simulink model "rlQubeServo"  (R2024a)
settings: Solver=ode23t  StartTime=0.0  StopTime=10.0  RelTol=1e-3  AbsTol=1e-3
values from neighbouring files (symbols this model uses):
  D_p = 8e-6    (= 8e-06)    [loadQubeParameters.m]
  D_r_2 = 1.88e-04    (= 0.000188)    [loadQubeParameters.m]
  dphi0 = 0    [loadQubeParameters.m]
  dphi_gain = 2    [loadQubeParameters.m]
  dtheta0 = 0    [loadQubeParameters.m]
  dtheta_gain = 0.0356    [loadQubeParameters.m]
  K_b_2 = 0.182    [loadQubeParameters.m]
  K_t = 0.042    [loadQubeParameters.m]
  L_m = 4.98e-3    (= 0.00498)    [loadQubeParameters.m]
  L_p = 0.126    [loadQubeParameters.m]
  L_r = 0.103    [loadQubeParameters.m]
  m_p = 0.024    [loadQubeParameters.m]
  m_r = 0.095    [loadQubeParameters.m]
  mu_m = 3.08e-6    (= 3.08e-06)    [loadQubeParameters.m]
  n = 1    [loadQubeParameters.m]
  p_rad = 0.0045    [loadQubeParameters.m]
  phi0 = 0    [loadQubeParameters.m]
  phi_gain = 40    [loadQubeParameters.m]
  R_m = 21.7    [loadQubeParameters.m]
  rod_rad = 0.003    [loadQubeParameters.m]
  Tf = 10    [loadQubeParameters.m]
  theta0 = 0    [loadQubeParameters.m]
  theta_gain = 0.162    [loadQubeParameters.m]
  Ts = Tc * 4    (= 0.02)    [loadQubeParameters.m]
  Volt_Limit = 12    [loadQubeParameters.m]
undefined symbols (not defined in the file or in its folder): X, Y, Z
libraries: sm_lib x21, fl_lib x10, nesl_utility x9, rllib x2, simulink x2, ee_lib x1
(part 1 of 2)
settings Model: Creator=The MathWorks, Inc.  LastModifiedBy=niels
settings SolverCC: AutoScaleAbsTol=off  MaxZcPerStep=1
settings DebuggingCC: UnconnectedInputMsg=warning  UnconnectedOutputMsg=warning  UnconnectedLineMsg=warning
settings ModelReferenceCC: EnableRefExpFcnMdlSchedulingChecks=on
settings RTWCC: GPUComputeCapability=3.5  DLArmComputeVersion=19.05
settings ExplorerConfigSet: InternalSimMechanicsExplorerSettings="<ExplorerConfiguration><canonicalview>default</canonicalview><AnimationSetting><BasePlaybackSpeed>1.0</BasePlaybackSpeed><PlaybackSpeedFactor>1.0</PlaybackSpeedFactor></AnimationSetting><TilePanel><TileInfo><Tiles Columns=\"1\" Count=\"1\" Rows=\"1\"><Column Weight=\"1\"/><Row Weight=\"1\"/><Tile Height=\"1\" Width=\"1\" X=\"0\" Y=\"0\"/></Tiles></TileInfo><SceneInfo><SceneViewer><BGColor><R>0.60000002384185791</R><G>0.60000002384185791</G><B>0.60000002384185791</B></BGColor><Camera><DoPerspective>on</DoPerspective><Position><X>0.334156231583514596</X><Y>0.107146061295956732</Y><Z>0.154419804164132285</Z></Position><Center><X>0.145480827141795971</X><Y>0.0537418892551446009</Y><Z>0.077934111254939889</Z></Center><Up><X>-0.332530024195597795</X><Y>-0.157027945704575345</Y><Z>0.929927958110882913</Z></Up><ViewLimDist>1</ViewLimDist><YLim>0.466307658154998583</YLim><XLim>0.535390274177961367</XLim></Camera></SceneViewer></SceneInfo></TilePanel><MechEditorPanel><Cameras><Camera><Id>Camera1</Id><Value><Name>Camera1</Name><NativeCamera><PositionKeyframeSet/><CenterKeyframeSet/><UpVectorKeyframeSet/></NativeCamera></Value></Camera></Cameras><GfxPanelCameraMap><MapElement CameraMLId=\"Camera1\" GfxPanelIndex=\"0\"/></GfxPanelCameraMap><VideoCreator><PlaybackSpeedRatio>1.0</PlaybackSpeedRatio><FrameRate>30</FrameRate><VideoFormat>Motion JPEG AVI</VideoFormat><FrameSize>auto</FrameSize></VideoCreator></MechEditorPanel></ExplorerConfiguration>"

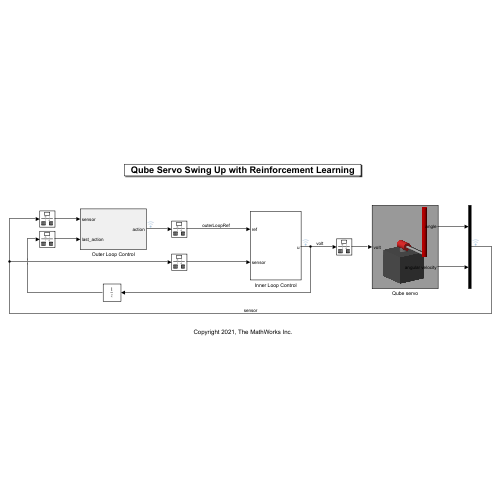
[thumbnail: Simulink's stored preview of the top-level diagram]
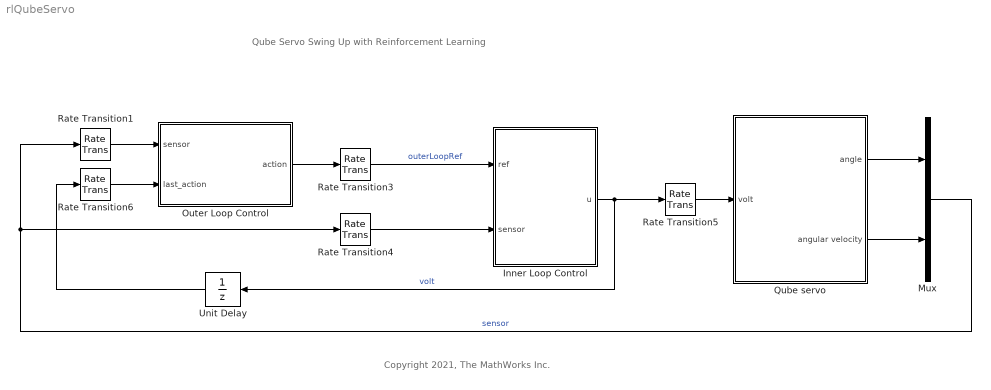
== system rlQubeServo ==
  note: Qube Servo Swing Up with Reinforcement Learning
  note: Copyright 2021, The MathWorks Inc.
  Inner Loop Control : Subsystem
  Mux : Mux  Inputs=2
  Outer Loop Control : Subsystem  mask{DesignModeChoice=Mode select}
      mask prompts: DesignModeChoice "Design mode"
      mask init:
      | choice = get_param(gcb,'DesignModeChoice');
      | vssBlk = [gcb,'/RL_Mode_Select/Variant Source'];
      | if strcmp(choice,'Swing up')
      |     set_param(vssBlk, 'LabelModeActiveChoice', 'RL_DESIGN_MODE_SWING_UP');
      | else
      |     set_param(vssBlk, 'LabelModeActiveChoice', 'RL_DESIGN_MODE_SELECT_MODE');
      | end
      mask TypeOptions DesignModeChoice: Mode select | Swing up
      mask DialogControl DescGroupVar Prompt: Description
      mask DialogControl DescTextVar Prompt: Select a design mode for the planner.
      mask DialogControl Control4 Prompt: A) Mode select:
      mask DialogControl Control2 Prompt: Select reference signal source for either pendulum swing up or balancing.
      mask DialogControl Control5 Prompt: B) Swing up:
      mask DialogControl Control3 Prompt: Swing up the pendulum from stable equilibrium position (phi=0 deg) without balancing
  Qube servo : Subsystem  mask(Qube servo 2 model by Simscape){a0=[theta0, phi0], w0=[dtheta0, dphi0], R_m=R_m, L_m=L_m, mu_m=mu_m, K_b=K_b_2, n=n, rod_mass=m_r, rod_length=L_r, rod_rad=rod_rad, p_mass=m_p, p_length=L_p, p_rad=p_rad, D_r=D_r_2, D_p=D_p, Choice_Stopper=Off}
      mask prompts: a0 "Init angle (theta phi) [rad]"; w0 "Init velocity (theta_dot phi_dot) [rad/s]"; R_m "Motor Resistance of [Ohm]"; L_m "Motor Inductance [H]"; mu_m "Motor Damping [Nm/rad/s]"; K_b "Back EMF contant [V/(rad/s)]"; n "Gear Ratio [-]"; rod_mass "Mass of Arm rod [kg]"; rod_length "Length of Arm rod [m]"; rod_rad "Radius of Arm rod [m]"; p_mass "Mass of Pendulum [kg]"; p_length "Length of Pendulum [m]"; p_rad "Radius of Pendulum [m]"; D_r "Damping of Arm rod [Nm/rad/s]"; D_p "Damping of Pendulum [Nm/rad/s]"; Choice_Stopper "Servo stopper"
      mask init:
      | % Density [kg/m^3] of each component
      | rho_rod = rod_mass/(pi*rod_rad^2*rod_length);
      | rho_p = p_mass/(pi*p_rad^2*p_length);
      | 
      | choice = get_param(gcb,'Choice_Stopper');
      | vssBlk = [gcb,'/Pendulum Physical Model/stopper'];
      | if strcmp(choice,'Off')
      |     set_param(vssBlk, 'LabelModeActiveChoice', 'Choice_Qube_Stopper_Off');
      | else
      |     set_param(vssBlk, 'LabelModeActiveChoice', 'Choice_Qube_Stopper_On');
      | end
      mask TypeOptions Choice_Stopper: Off | On
      mask DialogControl Container4 Prompt: Inital Conditions
      mask DialogControl Container3 Prompt: Parameters
      mask DialogControl Container7 Prompt: Options
      mask Display: image('$imagefile'); % Use "Edit Image" on toolstrip to change.
  Rate Transition1 : RateTransition  OutPortSampleTime=Ts
  Rate Transition3 : RateTransition  OutPortSampleTime=Tc
  Rate Transition4 : RateTransition  OutPortSampleTime=Tc
  Rate Transition5 : RateTransition
  Rate Transition6 : RateTransition  OutPortSampleTime=Ts
  Unit Delay : UnitDelay  SampleTime=-1  HasFrameUpgradeWarning=on
  wires:
  Qube servo/1(angle) -> Mux/1
  Qube servo/2(angular velocity) -> Mux/2
  Rate Transition4/1 -> Inner Loop Control/2(sensor)
  Inner Loop Control/1(u) -> Rate Transition5/1, Unit Delay/1  "volt"
  Rate Transition5/1 -> Qube servo/1(volt)
  Rate Transition3/1 -> Inner Loop Control/1(ref)  "outerLoopRef"
  Mux/1 -> Rate Transition1/1, Rate Transition4/1  "sensor"
  Unit Delay/1 -> Rate Transition6/1
  Rate Transition1/1 -> Outer Loop Control/1(sensor)
  Rate Transition6/1 -> Outer Loop Control/2(last_action)
  Outer Loop Control/1(action) -> Rate Transition3/1

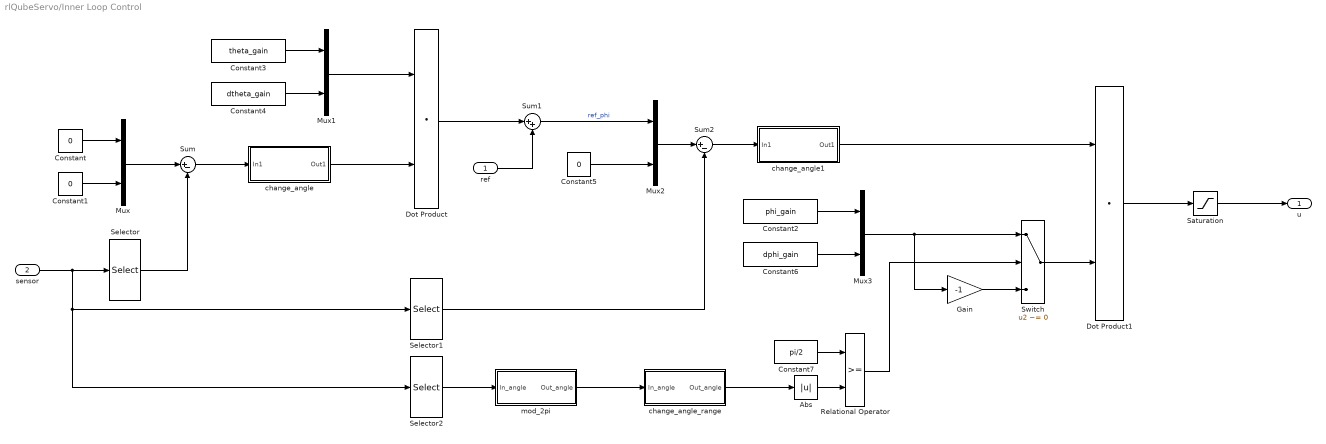
== system rlQubeServo/Inner Loop Control ==
  ref : Inport
  sensor : Inport  Port=2  PortDimensions=4
  Abs : Abs  SaturateOnIntegerOverflow=off
  Constant : Constant  Value=0
  Constant1 : Constant  Value=0
  Constant2 : Constant  Value=phi_gain
  Constant3 : Constant  Value=theta_gain
  Constant4 : Constant  Value=dtheta_gain
  Constant5 : Constant  Value=0
  Constant6 : Constant  Value=dphi_gain
  Constant7 : Constant  Value=pi/2
  Dot Product : DotProduct  OutDataTypeStr=Inherit: Inherit via internal rule
  Dot Product1 : DotProduct  OutDataTypeStr=Inherit: Inherit via internal rule
  Gain : Gain  Gain=-1
  Mux{,1..3} (4 alike) : Mux  Inputs=2
  Relational Operator : RelationalOperator  OutDataTypeStr=boolean  RndMeth=Simplest  InputSameDT=off
  Saturation : Saturate  UpperLimit=Volt_Limit  LowerLimit=-Volt_Limit
  Selector : Selector  InputPortWidth=4  IndexOptions=Index vector (dialog)  Indices=[1 3]  OutputSizes=1
  Selector1 : Selector  InputPortWidth=4  IndexOptions=Index vector (dialog)  Indices=[2 4]  OutputSizes=1
  Selector2 : Selector  InputPortWidth=4  IndexOptions=Index vector (dialog)  Indices=[2]  OutputSizes=1
  Sum : Sum  Inputs=|+-
  Sum1 : Sum  Inputs=|++
  Sum2 : Sum  Inputs=|+-
  Switch : Switch  Criteria=u2 ~= 0  SaturateOnIntegerOverflow=off  InputSameDT=off
  change_angle : Subsystem
  change_angle1 : Subsystem
  change_angle_range : Subsystem
  mod_2pi : Subsystem
  u : Outport
  wires:
  change_angle_range/1(Out_angle) -> Abs/1
  Constant4/1 -> Mux1/2
  Constant2/1 -> Mux3/1
  Saturation/1 -> u/1
  Relational Operator/1 -> Switch/2
  Gain/1 -> Switch/3
  Constant7/1 -> Relational Operator/1
  sensor/1 -> Selector2/1, Selector1/1, Selector/1
  Sum/1 -> change_angle/1(In1)
  ref/1 -> Sum1/2
  Selector1/1 -> Sum2/2
  Selector2/1 -> mod_2pi/1(In_angle)
  Dot Product1/1 -> Saturation/1
  Sum2/1 -> change_angle1/1(In1)
  Constant5/1 -> Mux2/2
  Constant6/1 -> Mux3/2
  Mux2/1 -> Sum2/1
  Abs/1 -> Relational Operator/2
  mod_2pi/1(Out_angle) -> change_angle_range/1(In_angle)
  Sum1/1 -> Mux2/1  "ref_phi"
  Mux1/1 -> Dot Product/1
  Constant3/1 -> Mux1/1
  change_angle1/1(Out1) -> Dot Product1/1
  Constant/1 -> Mux/1
  Dot Product/1 -> Sum1/1
  Mux/1 -> Sum/1
  Mux3/1 -> Switch/1, Gain/1
  Switch/1 -> Dot Product1/2
  Constant1/1 -> Mux/2
  change_angle/1(Out1) -> Dot Product/2
  Selector/1 -> Sum/2

== system rlQubeServo/Outer Loop Control ==
  sensor : Inport
  last_action : Inport  Port=2
  RL_Mode_Select : Subsystem
  RL_Swing_Up : Subsystem
  Switch_Action : Subsystem
  action : Outport
  wires:
  RL_Swing_Up/1(swing_up) -> Switch_Action/2(swing_up)  "action_RL_swing_up"
  Switch_Action/1(out_action) -> action/1  "action"
  sensor/1 -> RL_Swing_Up/1(sensor), RL_Mode_Select/1(sensor)
  RL_Mode_Select/1(select_mode) -> Switch_Action/1(select_mode)  "action_RL_select_mode"
  last_action/1 -> RL_Mode_Select/2(controller_action), RL_Swing_Up/2(controller_action)

== system rlQubeServo/Qube servo ==
  volt : Inport
  DC Motor model : Subsystem
  Pendulum Physical Model : Subsystem
  Terminator1 : Terminator
  angle : Outport
  angular velocity : Outport  Port=2
  wires:
  Pendulum Physical Model/3(Load trq) -> Terminator1/1
  Pendulum Physical Model/1(angle) -> angle/1
  volt/1 -> DC Motor model/1(volt)
  Pendulum Physical Model/2(velocity) -> angular velocity/1
  connections:
  DC Motor model/RConn2 -- Pendulum Physical Model/LConn2
  DC Motor model/RConn1 -- Pendulum Physical Model/LConn1

== system rlQubeServo/Inner Loop Control/change_angle ==
  In1 : Inport
  Demux : Demux  Outputs=2
  Mux : Mux  Inputs=2
  change_angle_range : Subsystem
  mod_2pi : Subsystem
  Out1 : Outport
  wires:
  In1/1 -> Demux/1
  Demux/1 -> mod_2pi/1(In_angle)
  mod_2pi/1(Out_angle) -> change_angle_range/1(In_angle)
  change_angle_range/1(Out_angle) -> Mux/1
  Demux/2 -> Mux/2
  Mux/1 -> Out1/1

== system rlQubeServo/Inner Loop Control/change_angle1 ==
  In1 : Inport
  Demux : Demux  Outputs=2
  Mux : Mux  Inputs=2
  change_angle_range : Subsystem
  mod_2pi : Subsystem
  Out1 : Outport
  wires:
  Mux/1 -> Out1/1
  Demux/2 -> Mux/2
  change_angle_range/1(Out_angle) -> Mux/1
  mod_2pi/1(Out_angle) -> change_angle_range/1(In_angle)
  Demux/1 -> mod_2pi/1(In_angle)
  In1/1 -> Demux/1

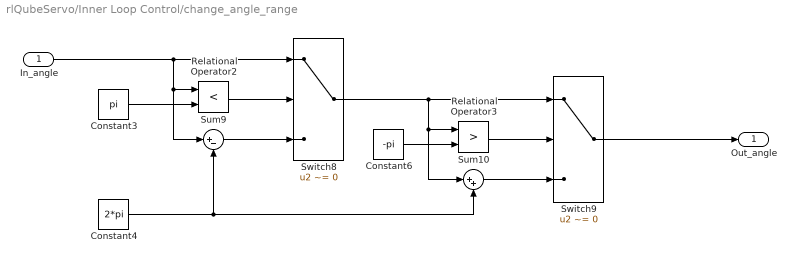
== system rlQubeServo/Inner Loop Control/change_angle_range ==
  In_angle : Inport
  Constant3 : Constant  Value=pi  OutDataTypeStr=Inherit: Inherit via back propagation
  Constant4 : Constant  Value=2*pi  OutDataTypeStr=Inherit: Inherit via back propagation
  Constant6 : Constant  Value=-pi  OutDataTypeStr=Inherit: Inherit via back propagation
  Relational Operator2 : RelationalOperator  Operator=<  OutDataTypeStr=boolean  InputSameDT=off
  Relational Operator3 : RelationalOperator  Operator=>  OutDataTypeStr=boolean  InputSameDT=off
  Sum10 : Sum  Inputs=|++
  Sum9 : Sum  Inputs=|+-
  Switch8 : Switch  Criteria=u2 ~= 0  SaturateOnIntegerOverflow=off  InputSameDT=off
  Switch9 : Switch  Criteria=u2 ~= 0  SaturateOnIntegerOverflow=off  InputSameDT=off
  Out_angle : Outport
  wires:
  Switch9/1 -> Out_angle/1
  Sum9/1 -> Switch8/3
  Switch8/1 -> Relational Operator3/1, Sum10/1, Switch9/1
  Constant6/1 -> Relational Operator3/2
  Constant4/1 -> Sum10/2, Sum9/2
  Relational Operator3/1 -> Switch9/2
  Constant3/1 -> Relational Operator2/2
  Sum10/1 -> Switch9/3
  Relational Operator2/1 -> Switch8/2
  In_angle/1 -> Relational Operator2/1, Sum9/1, Switch8/1

== system rlQubeServo/Inner Loop Control/mod_2pi ==
  In_angle : Inport
  MATLAB Function : MATLAB Function  TreatAsAtomicUnit=on
  Out_angle : Outport
  wires:
  MATLAB Function/1(y) -> Out_angle/1
  In_angle/1 -> MATLAB Function/1(u)

== system rlQubeServo/Outer Loop Control/RL_Mode_Select ==
  sensor : Inport
  controller_action : Inport  Port=2
  Constant : Constant  Value=0
  RL_agent_select_mode : rllib/RL Agent  Agent=modeAgent  ExternalActionAsInput=off  ProvideLastAction=off  ProvideCumRwd=off  TreatAsDirectFeedthrough=on  UseStrictObservationDataTypes=off
  Variant Source : VariantSource  VariantControlMode=label  LabelModeActiveChoice=RL_DESIGN_MODE_SELECT_MODE
  isdone : Subsystem  VariantControl=VARIANT_INV_POS
  "observation " : Subsystem  VariantControl=VARIANT_OBS_ARM_PEND
  reward : Subsystem  VariantControl=VARIANT_INV_POS
  select_mode : Outport
  wires:
  RL_agent_select_mode/1 -> Variant Source/2
  "observation "/1(observation) -> RL_agent_select_mode/1  "observation_select_mode"
  reward/1(reward) -> RL_agent_select_mode/2  "reward_select_mode"
  controller_action/1 -> reward/2(action)
  isdone/2(isdone_flag_delay) -> RL_agent_select_mode/3  "isdone_select_mode"
  sensor/1 -> "observation "/1(sensor), isdone/1(sensor), reward/1(sensor)
  isdone/1(isdone_flag) -> reward/3(isdone_flag)
  Variant Source/1 -> select_mode/1
  Constant/1 -> Variant Source/1

== system rlQubeServo/Outer Loop Control/RL_Swing_Up ==
  sensor : Inport
  controller_action : Inport  Port=2
  Gain : Gain  Gain=3*pi/4
  RL_agent_swing_up : rllib/RL Agent  Agent=swingAgent  ExternalActionAsInput=off  ProvideLastAction=off  ProvideCumRwd=off  TreatAsDirectFeedthrough=on  UseStrictObservationDataTypes=off
  isdone : Subsystem  VariantControl=VARIANT_INV_POS
  "observation " : Subsystem  VariantControl=VARIANT_OBS_ARM_PEND
  reward : Subsystem  VariantControl=VARIANT_INV_POS
  swing_up : Outport
  wires:
  isdone/1(isdone_flag) -> reward/3(isdone_flag)
  sensor/1 -> "observation "/1(sensor), isdone/1(sensor), reward/1(sensor)
  isdone/2(isdone_flag_delay) -> RL_agent_swing_up/3  "isdone_swing_up"
  controller_action/1 -> reward/2(action)
  reward/1(reward) -> RL_agent_swing_up/2  "reward_swing_up"
  "observation "/1(observation) -> RL_agent_swing_up/1  "observation_swing_up"
  RL_agent_swing_up/1 -> Gain/1
  Gain/1 -> swing_up/1

== system rlQubeServo/Outer Loop Control/Switch_Action ==
  select_mode : Inport
  swing_up : Inport  Port=2
  Constant : Constant  Value=pi
  Constant1 : Constant  OutDataTypeStr=int32
  Data Type Conversion : DataTypeConversion  OutDataTypeStr=int32  SaturateOnIntegerOverflow=off  RndMeth=Floor
  Relational Operator : RelationalOperator  Operator===  OutDataTypeStr=boolean  RndMeth=Simplest  InputSameDT=off
  Switch : Switch  Criteria=u2 > Threshold  SaturateOnIntegerOverflow=off  InputSameDT=off
  out_action : Outport
  wires:
  Constant/1 -> Switch/1
  swing_up/1 -> Switch/3
  Constant1/1 -> Relational Operator/1
  Switch/1 -> out_action/1
  select_mode/1 -> Data Type Conversion/1
  Relational Operator/1 -> Switch/2
  Data Type Conversion/1 -> Relational Operator/2

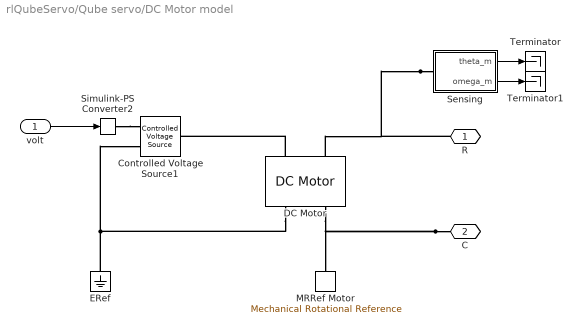
== system rlQubeServo/Qube servo/DC Motor model ==
  volt : Inport
  Controlled Voltage Source1 : fl_lib/Electrical/Electrical Sources/Controlled Voltage Source
  DC Motor : ee_lib/Electromechanical/Brushed Motors/DC Motor  field_option=ee.enum.field_option.pm  Rf=100 Ohm  Lf=1 H  Laf=0.15 H  If0=0 A  parameterization=ee.enum.dcparam_option.circuit_param  Ra=R_m Ohm  La=L_m H  emf_or_torque=ee.enum.emf_or_torque.kv  Kv=K_b V/(rad/s)  Ki=K_t N*m/A  T_stall=0.24e-3 N*m  w_max=19100 rpm  w_rated=15000 rpm  P_rated=0.08 W  V_rated=1.5 V  lam_param=ee.enum.lam_param.damping  i_noload=0 A  V_i_noload=1.5 V  J=0 g*cm^2  lam=0 N*m/(rad/s)  speed0=0 rpm  enable_fault_armature=simscape.enum.onoff.off  rev_faulted=1 / 3  G_faulted_armature=1e-5 S  fault_trigger_armature=ee.enum.faults.faultTrigger.temporal  t_fault_armature=1 s  max_permissible_current_armature=inf A  t_fail_on_current_armature=1 s  enable_fault_field=simscape.enum.onoff.off  G_faulted_field=1e-5 S  fault_trigger_field=ee.enum.faults.faultTrigger.temporal  t_fault_field=1 s  max_permissible_current_field=inf A  t_fail_on_current_field=1 s  fault_action=simscape.enum.assert.action.none  alpha=3.93e-3 1/K  Tmeas=25 degC  thermal_mass=100 J/K  initial_temperature=25 degC
  ERef : fl_lib/Electrical/Electrical Elements/Electrical Reference
  MRRef Motor : fl_lib/Mechanical/Rotational Elements/Mechanical Rotational Reference
  Sensing : Subsystem
  Simulink-PS Converter2 : nesl_utility/Simulink-PS Converter  PhysicalDomain=network_engine_domain  SubClassName=ps_input  LeftPortType=input  RightPortType=output  PseudoPeriodic=off  Frequencies=[]  NoiseDistribution=none  NoiseParameters=[]  Unit=1  AffineConversion=off  FilteringAndDerivatives=provide  SimscapeFilterOrder=1  InputFilterTimeConstant=0.001  UdotUserProvided=0
  Terminator : Terminator
  Terminator1 : Terminator
  R : PMIOPort  Side=Right
  C : PMIOPort  Port=2  Side=Right
  wires:
  Sensing/2(omega_m) -> Terminator1/1
  Sensing/1(theta_m) -> Terminator/1
  volt/1 -> Simulink-PS Converter2/1
  connections:
  DC Motor/LConn1 -- Controlled Voltage Source1/LConn1
  Sensing/LConn1 -- DC Motor/LConn2 -- R/RConn1
  Simulink-PS Converter2/RConn1 -- Controlled Voltage Source1/RConn1
  ERef/LConn1 -- DC Motor/RConn1 -- Controlled Voltage Source1/RConn2
  C/RConn1 -- DC Motor/RConn2 -- MRRef Motor/LConn1

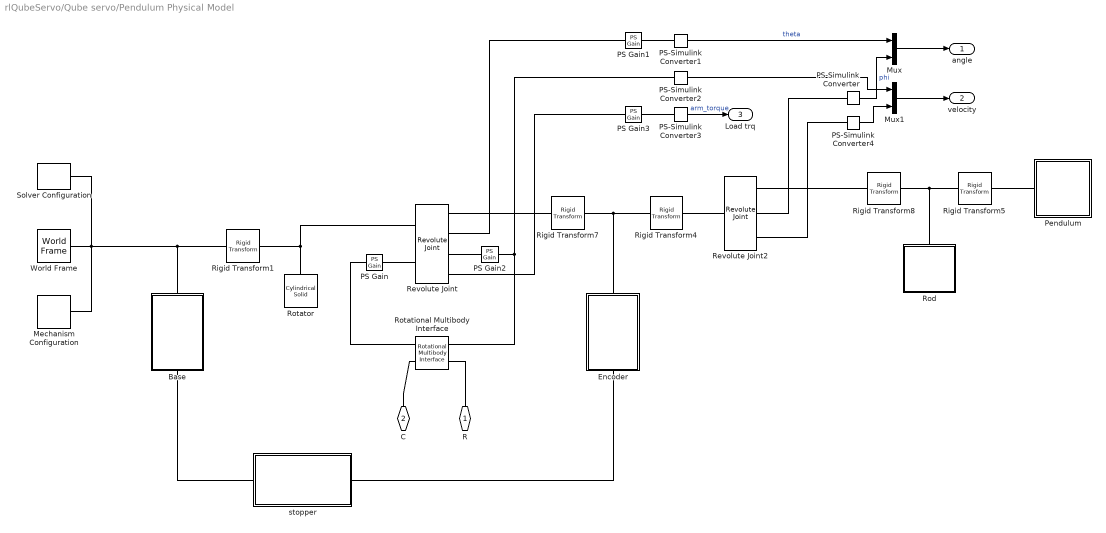
== system rlQubeServo/Qube servo/Pendulum Physical Model ==
  Base : Subsystem
  Encoder : Subsystem
  Mechanism Configuration : sm_lib/Utilities/Mechanism Configuration  UniformGravity=Constant  GravityVector=[0 0 -9.80665]  GravityVectorUnits=m/s^2  LinearizationDelta=0.001  JointModeTransitionNonlinearIterations=2
  Mux : Mux  Inputs=2
  Mux1 : Mux  Inputs=2
  PS Gain{,1..3} (4 alike) : fl_lib/Physical Signals/Functions/PS Gain  gain=-1
  PS-Simulink Converter{,1..4} (5 alike) : nesl_utility/PS-Simulink Converter  PhysicalDomain=network_engine_domain  SubClassName=ps_output  LeftPortType=input  RightPortType=output  PseudoPeriodic=off  Frequencies=[]  VectorFormat=1-D array  Unit=inherit  AffineConversion=off
  Pendulum : Subsystem
  Revolute Joint : sm_lib/Joints/Revolute Joint  JointMode=Normal  CompositeWrenchDir=FollowerOnBase  CompositeWrenchFrame=BaseFrame  SenseConstraintForce=off  SenseConstraintTorque=off  SenseTotalForce=off  SenseTotalTorque=off  PositionTargetSpecify=on  PositionTargetPriority=High  PositionTargetValue=a0(1)  PositionTargetValueUnits=rad  VelocityTargetSpecify=off  VelocityTargetPriority=High  VelocityTargetValue=0  VelocityTargetValueUnits=deg/s  EquilibriumPosition=0  EquilibriumPositionUnits=deg  SpringStiffness=0  SpringStiffnessUnits=N*m/deg  DampingCoefficient=D_r  DampingCoefficientUnits=N*m/(rad/s)  LowerLimitSpecify=off  LowerLimitBound=-90  LowerLimitBoundUnits=deg  LowerLimitStiffness=1e4  LowerLimitStiffnessUnits=N*m/deg  LowerLimitDamping=10  LowerLimitDampingUnits=N*m/(deg/s)  LowerLimitTransitionRegionWidth=0.1  LowerLimitTransitionRegionWidthUnits=deg  UpperLimitSpecify=off  UpperLimitBound=90  UpperLimitBoundUnits=deg  UpperLimitStiffness=1e4  UpperLimitStiffnessUnits=N*m/deg  UpperLimitDamping=10  UpperLimitDampingUnits=N*m/(deg/s)  UpperLimitTransitionRegionWidth=0.1  UpperLimitTransitionRegionWidthUnits=deg  TorqueActuationMode=InputTorque  MotionActuationMode=ComputedMotion  SensePosition=on  SenseVelocity=on  SenseAcceleration=off  SenseTorqueForce=on  SenseLowerLimitTorqueForce=off  SenseUpperLimitTorqueForce=off
  Revolute Joint2 : sm_lib/Joints/Revolute Joint  JointMode=Normal  CompositeWrenchDir=FollowerOnBase  CompositeWrenchFrame=BaseFrame  SenseConstraintForce=off  SenseConstraintTorque=off  SenseTotalForce=off  SenseTotalTorque=off  PositionTargetSpecify=on  PositionTargetPriority=High  PositionTargetValue=a0(2)  PositionTargetValueUnits=rad  VelocityTargetSpecify=off  VelocityTargetPriority=High  VelocityTargetValue=0  VelocityTargetValueUnits=deg/s  EquilibriumPosition=0  EquilibriumPositionUnits=deg  SpringStiffness=0  SpringStiffnessUnits=N*m/deg  DampingCoefficient=D_p  DampingCoefficientUnits=N*m/(rad/s)  LowerLimitSpecify=off  LowerLimitBound=-90  LowerLimitBoundUnits=deg  LowerLimitStiffness=1e4  LowerLimitStiffnessUnits=N*m/deg  LowerLimitDamping=10  LowerLimitDampingUnits=N*m/(deg/s)  LowerLimitTransitionRegionWidth=0.1  LowerLimitTransitionRegionWidthUnits=deg  UpperLimitSpecify=off  UpperLimitBound=90  UpperLimitBoundUnits=deg  UpperLimitStiffness=1e4  UpperLimitStiffnessUnits=N*m/deg  UpperLimitDamping=10  UpperLimitDampingUnits=N*m/(deg/s)  UpperLimitTransitionRegionWidth=0.1  UpperLimitTransitionRegionWidthUnits=deg  TorqueActuationMode=NoTorque  MotionActuationMode=ComputedMotion  SensePosition=on  SenseVelocity=on  SenseAcceleration=off  SenseTorqueForce=off  SenseLowerLimitTorqueForce=off  SenseUpperLimitTorqueForce=off
  Rigid Transform1 : sm_lib/Frames and Transforms/Rigid Transform  RotationMethod=None  FollAlignAxisA=+X  BaseAlignAxisA=+Y  FollAlignAxisB=+Y  BaseAlignAxisB=+Z  RotationStandardAxis=+Y  RotationAngle=90  RotationAngleUnits=deg  RotationArbitraryAxis=[0 0 1]  RotationSequenceAxes=FollowerAxes  RotationSequence=XYX  RotationSequenceAngles=[0 0 0]  RotationSequenceAnglesUnits=deg  RotationMatrix=[1 0 0; 0 1 0; 0 0 1]  Quaternion=[1 0 0 0]  TranslationMethod=Cartesian  TranslationCartesianOffset=[0 0 5]  TranslationCartesianOffsetUnits=cm  TranslationStandardAxis=+Z  TranslationStandardOffset=0  TranslationStandardOffsetUnits=cm  TranslationROffset=0  TranslationROffsetUnits=m  TranslationThetaOffset=0  TranslationThetaOffsetUnits=deg  TranslationZOffset=0  TranslationZOffsetUnits=m
  Rigid Transform4 : sm_lib/Frames and Transforms/Rigid Transform  RotationMethod=StandardAxis  FollAlignAxisA=+X  BaseAlignAxisA=+Y  FollAlignAxisB=+Y  BaseAlignAxisB=+Z  RotationStandardAxis=+Y  RotationAngle=90  RotationAngleUnits=deg  RotationArbitraryAxis=[0 0 1]  RotationSequenceAxes=FollowerAxes  RotationSequence=XYX  RotationSequenceAngles=[0 0 0]  RotationSequenceAnglesUnits=deg  RotationMatrix=[1 0 0; 0 1 0; 0 0 1]  Quaternion=[1 0 0 0]  TranslationMethod=None  TranslationCartesianOffset=[-1.3 1 0]  TranslationCartesianOffsetUnits=cm  TranslationStandardAxis=+Z  TranslationStandardOffset=0  TranslationStandardOffsetUnits=cm  TranslationROffset=0  TranslationROffsetUnits=m  TranslationThetaOffset=0  TranslationThetaOffsetUnits=deg  TranslationZOffset=0  TranslationZOffsetUnits=m
  Rigid Transform5 : sm_lib/Frames and Transforms/Rigid Transform  RotationMethod=AlignedAxes  FollAlignAxisA=+X  BaseAlignAxisA=+Z  FollAlignAxisB=+Z  BaseAlignAxisB=+X  RotationStandardAxis=+Y  RotationAngle=90  RotationAngleUnits=deg  RotationArbitraryAxis=[0 0 1]  RotationSequenceAxes=FollowerAxes  RotationSequence=XYX  RotationSequenceAngles=[0 0 0]  RotationSequenceAnglesUnits=deg  RotationMatrix=[1 0 0; 0 1 0; 0 0 1]  Quaternion=[1 0 0 0]  TranslationMethod=StandardAxis  TranslationCartesianOffset=[0 0 0]  TranslationCartesianOffsetUnits=m  TranslationStandardAxis=+Z  TranslationStandardOffset=rod_length/2  TranslationStandardOffsetUnits=m  TranslationROffset=0  TranslationROffsetUnits=m  TranslationThetaOffset=0  TranslationThetaOffsetUnits=deg  TranslationZOffset=0  TranslationZOffsetUnits=m
  Rigid Transform7 : sm_lib/Frames and Transforms/Rigid Transform  RotationMethod=None  FollAlignAxisA=+X  BaseAlignAxisA=+Y  FollAlignAxisB=+Y  BaseAlignAxisB=+Z  RotationStandardAxis=+X  RotationAngle=90  RotationAngleUnits=deg  RotationArbitraryAxis=[0 0 1]  RotationSequenceAxes=FollowerAxes  RotationSequence=XYX  RotationSequenceAngles=[0 0 0]  RotationSequenceAnglesUnits=deg  RotationMatrix=[1 0 0; 0 1 0; 0 0 1]  Quaternion=[1 0 0 0]  TranslationMethod=Cartesian  TranslationCartesianOffset=[0 0 2]  TranslationCartesianOffsetUnits=cm  TranslationStandardAxis=+Z  TranslationStandardOffset=0  TranslationStandardOffsetUnits=cm  TranslationROffset=0  TranslationROffsetUnits=m  TranslationThetaOffset=0  TranslationThetaOffsetUnits=deg  TranslationZOffset=0  TranslationZOffsetUnits=m
  Rigid Transform8 : sm_lib/Frames and Transforms/Rigid Transform  RotationMethod=None  FollAlignAxisA=+X  BaseAlignAxisA=+Y  FollAlignAxisB=+Y  BaseAlignAxisB=+Z  RotationStandardAxis=+Y  RotationAngle=-90  RotationAngleUnits=deg  RotationArbitraryAxis=[0 0 1]  RotationSequenceAxes=FollowerAxes  RotationSequence=XYX  RotationSequenceAngles=[0 0 0]  RotationSequenceAnglesUnits=deg  RotationMatrix=[1 0 0; 0 1 0; 0 0 1]  Quaternion=[1 0 0 0]  TranslationMethod=Cartesian  TranslationCartesianOffset=[0 0 (rod_length/2 - 0.018)]  TranslationCartesianOffsetUnits=m  TranslationStandardAxis=+Z  TranslationStandardOffset=0  TranslationStandardOffsetUnits=m  TranslationROffset=0  TranslationROffsetUnits=m  TranslationThetaOffset=0  TranslationThetaOffsetUnits=deg  TranslationZOffset=0  TranslationZOffsetUnits=m
  Rod : Subsystem
  Rotational Multibody Interface : fl_lib/Mechanical/Multibody Interfaces/Rotational Multibody Interface
  Rotator : sm_lib/Body Elements/Cylindrical Solid  CylinderRadius=1  CylinderRadiusUnits=cm  CylinderLength=3  CylinderLengthUnits=cm  ExportEntireGeometry=off  InertiaType=PointMass  BasedOnType=Density  Density=1000  DensityUnits=kg/m^3  Mass=0  MassUnits=kg  CenterOfMass=[0 0 0]  CenterOfMassUnits=m  MomentsOfInertia=[1 1 1]  MomentsOfInertiaUnits=kg*m^2  ProductsOfInertia=[0 0 0]  ProductsOfInertiaUnits=kg*m^2  GraphicType=FromGeometry  MarkerShape=Sphere  MarkerSize=10  GraphicVisPropType=SimpleVisualProperties  GraphicDiffuseColor=[0.6 0.6 0.6]  GraphicOpacity=1.0  GraphicSpecularColor=[0.5 0.5 0.5 1.0]  GraphicAmbientColor=[0.15 0.15 0.15 1.0]  GraphicEmissiveColor=[0.0 0.0 0.0 1.0]  GraphicShininess=75  DoExposeReferenceFrame=on  SerializedFrames=<Frames/>
  Solver Configuration : nesl_utility/Solver Configuration  PhysicalDomain=network_engine_domain  SubClassName=solver  LeftPortType=input  RightPortType=generic  Tones=[]  Harmonics=[]  SimulateNoise=off  Profile=off  UseLocalSampling=off  EnableSwitchedLinearOptims=on  FrequencyDomain=off  UseCCode=off  RelTol=0.001  AbsTol=1e-06  MinStep=1e-09  ToWorkspace=off  RevertToSquareIcSolve=off  NumHomotopyIterations=100  PhasorMode=off  PhasorModeNumHarmonics=1  ConsistencySolver=NEWTON_FTOL  IndexReductionMethod=DerivativeReplacement  DoDC=off  ResidualTolerance=1e-09  ConsistencyTolSource=GLOBAL  ConsistencyAbsTol=0.001  ConsistencyRelTol=0.001  ConsistencyTolFactor=0.001  UseLocalSolver=off  LocalSolverChoice=NE_BACKWARD_EULER_ADVANCER  ResolveIndetEquations=on  FunctionEvalNumThread=1  LocalSolverSampleTime=0.001  DoFixedCost=off  MaxNonlinIter=3  MaxModeIter=2  ComputeImpulses=off  ImpulseIterations=2  LinearAlgebra=Sparse  LinearAlgebraNumThread=0  EquationFormulation=NE_TIME_EF  DelaysMemoryBudget=1024  AutomaticFiltering=on  FilteringTimeConstant=0.001  PartitionStorageMethod=AS_NEEDED  PartitionMemoryBudget=1024  PartitionMethod=FAST  MultibodyUseLocalSolver=off  MultibodyLocalSolverChoice=ODE1  MultibodyLocalSolverSampleTime=0.001
  World Frame : sm_lib/Frames and Transforms/World Frame
  stopper : Subsystem  Variant=on  VariantControlMode=label  VariantControl=Choice  LabelModeActiveChoice=Choice_Qube_Stopper_Off
  R : PMIOPort  Side=Left
  C : PMIOPort  Port=2  Side=Left
  angle : Outport
  velocity : Outport  Port=2
  Load trq : Outport  Port=3
  wires:
  Mux/1 -> angle/1
  Mux1/1 -> velocity/1
  PS-Simulink Converter4/1 -> Mux1/2
  PS-Simulink Converter/1 -> Mux/2  "phi"
  PS-Simulink Converter1/1 -> Mux/1  "theta"
  PS-Simulink Converter3/1 -> Load trq/1  "arm_torque"
  PS-Simulink Converter2/1 -> Mux1/1
  connections:
  Rotator/RConn1 -- Revolute Joint/LConn1 -- Rigid Transform1/RConn1
  Revolute Joint2/RConn3 -- PS-Simulink Converter4/LConn1
  C/RConn1 -- Rotational Multibody Interface/LConn2
  Rotational Multibody Interface/RConn2 -- R/RConn1
  Rotational Multibody Interface/LConn1 -- PS Gain/LConn1
  Revolute Joint/RConn4 -- PS Gain3/LConn1
  PS-Simulink Converter1/LConn1 -- PS Gain1/RConn1
  Revolute Joint2/RConn1 -- Rigid Transform8/LConn1
  World Frame/RConn1 -- Solver Configuration/RConn1 -- Rigid Transform1/LConn1 -- Base/RConn1 -- Mechanism Configuration/RConn1
  Rigid Transform4/RConn1 -- Revolute Joint2/LConn1
  Rigid Transform4/LConn1 -- Rigid Transform7/RConn1 -- Encoder/LConn1
  Revolute Joint/RConn1 -- Rigid Transform7/LConn1
  PS-Simulink Converter/LConn1 -- Revolute Joint2/RConn2
  Pendulum/LConn1 -- Rigid Transform5/RConn1
  PS-Simulink Converter2/LConn1 -- Rotational Multibody Interface/RConn1 -- PS Gain2/RConn1
  stopper/LConn1 -- Base/LConn1
  stopper/RConn1 -- Encoder/RConn1
  PS Gain/RConn1 -- Revolute Joint/LConn2
  PS Gain1/LConn1 -- Revolute Joint/RConn2
  PS Gain3/RConn1 -- PS-Simulink Converter3/LConn1
  Revolute Joint/RConn3 -- PS Gain2/LConn1
  Rigid Transform8/RConn1 -- Rigid Transform5/LConn1 -- Rod/LConn1

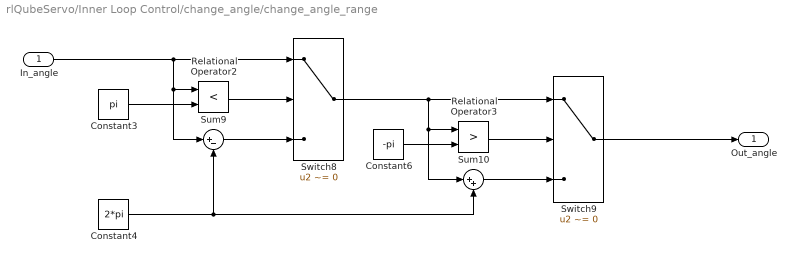
== system rlQubeServo/Inner Loop Control/change_angle/change_angle_range ==
  In_angle : Inport
  Constant3 : Constant  Value=pi  OutDataTypeStr=Inherit: Inherit via back propagation
  Constant4 : Constant  Value=2*pi  OutDataTypeStr=Inherit: Inherit via back propagation
  Constant6 : Constant  Value=-pi  OutDataTypeStr=Inherit: Inherit via back propagation
  Relational Operator2 : RelationalOperator  Operator=<  OutDataTypeStr=boolean  InputSameDT=off
  Relational Operator3 : RelationalOperator  Operator=>  OutDataTypeStr=boolean  InputSameDT=off
  Sum10 : Sum  Inputs=|++
  Sum9 : Sum  Inputs=|+-
  Switch8 : Switch  Criteria=u2 ~= 0  SaturateOnIntegerOverflow=off  InputSameDT=off
  Switch9 : Switch  Criteria=u2 ~= 0  SaturateOnIntegerOverflow=off  InputSameDT=off
  Out_angle : Outport
  wires:
  Switch9/1 -> Out_angle/1
  Sum9/1 -> Switch8/3
  Switch8/1 -> Relational Operator3/1, Sum10/1, Switch9/1
  Constant6/1 -> Relational Operator3/2
  Constant4/1 -> Sum10/2, Sum9/2
  Relational Operator3/1 -> Switch9/2
  Constant3/1 -> Relational Operator2/2
  Sum10/1 -> Switch9/3
  Relational Operator2/1 -> Switch8/2
  In_angle/1 -> Relational Operator2/1, Sum9/1, Switch8/1

== system rlQubeServo/Inner Loop Control/change_angle/mod_2pi ==
  In_angle : Inport
  MATLAB Function : MATLAB Function  TreatAsAtomicUnit=on
  Out_angle : Outport
  wires:
  MATLAB Function/1(y) -> Out_angle/1
  In_angle/1 -> MATLAB Function/1(u)

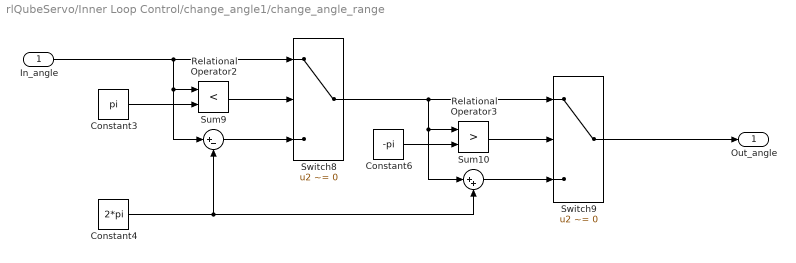
== system rlQubeServo/Inner Loop Control/change_angle1/change_angle_range ==
  In_angle : Inport
  Constant3 : Constant  Value=pi  OutDataTypeStr=Inherit: Inherit via back propagation
  Constant4 : Constant  Value=2*pi  OutDataTypeStr=Inherit: Inherit via back propagation
  Constant6 : Constant  Value=-pi  OutDataTypeStr=Inherit: Inherit via back propagation
  Relational Operator2 : RelationalOperator  Operator=<  OutDataTypeStr=boolean  InputSameDT=off
  Relational Operator3 : RelationalOperator  Operator=>  OutDataTypeStr=boolean  InputSameDT=off
  Sum10 : Sum  Inputs=|++
  Sum9 : Sum  Inputs=|+-
  Switch8 : Switch  Criteria=u2 ~= 0  SaturateOnIntegerOverflow=off  InputSameDT=off
  Switch9 : Switch  Criteria=u2 ~= 0  SaturateOnIntegerOverflow=off  InputSameDT=off
  Out_angle : Outport
  wires:
  Switch9/1 -> Out_angle/1
  Sum9/1 -> Switch8/3
  Switch8/1 -> Relational Operator3/1, Sum10/1, Switch9/1
  Constant6/1 -> Relational Operator3/2
  Constant4/1 -> Sum10/2, Sum9/2
  Relational Operator3/1 -> Switch9/2
  Constant3/1 -> Relational Operator2/2
  Sum10/1 -> Switch9/3
  Relational Operator2/1 -> Switch8/2
  In_angle/1 -> Relational Operator2/1, Sum9/1, Switch8/1

== system rlQubeServo/Inner Loop Control/change_angle1/mod_2pi ==
  In_angle : Inport
  MATLAB Function : MATLAB Function  TreatAsAtomicUnit=on
  Out_angle : Outport
  wires:
  MATLAB Function/1(y) -> Out_angle/1
  In_angle/1 -> MATLAB Function/1(u)

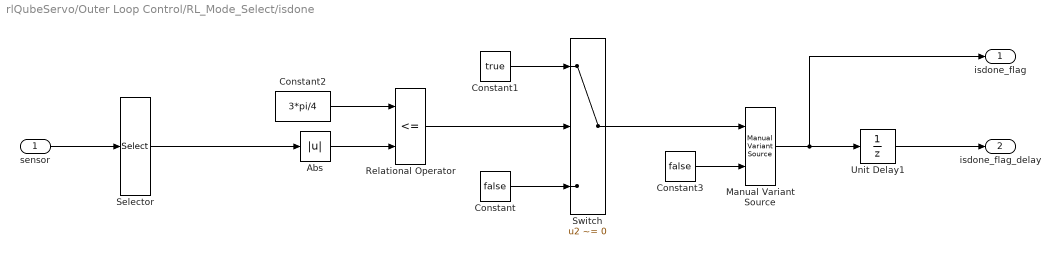
== system rlQubeServo/Outer Loop Control/RL_Mode_Select/isdone ==
  sensor : Inport
  Abs : Abs  SaturateOnIntegerOverflow=off
  Constant : Constant  Value=false
  Constant1 : Constant  Value=true
  Constant2 : Constant  Value=3*pi/4
  Constant3 : Constant  Value=false
  Manual Variant Source : simulink/Signal Routing/Manual Variant Source  NumChoices=2  LabelModeActiveChoice=V_2
  Relational Operator : RelationalOperator  Operator=<=  OutDataTypeStr=boolean  RndMeth=Simplest  InputSameDT=off
  Selector : Selector  InputPortWidth=4  IndexOptions=Index vector (dialog)  Indices=[1]  OutputSizes=1
  Switch : Switch  Criteria=u2 ~= 0  SaturateOnIntegerOverflow=off  InputSameDT=off
  Unit Delay1 : UnitDelay  SampleTime=-1  HasFrameUpgradeWarning=on
  isdone_flag : Outport
  isdone_flag_delay : Outport  Port=2
  wires:
  Unit Delay1/1 -> isdone_flag_delay/1
  Constant3/1 -> Manual Variant Source/2
  Manual Variant Source/1 -> Unit Delay1/1, isdone_flag/1
  Switch/1 -> Manual Variant Source/1
  Selector/1 -> Abs/1
  Constant1/1 -> Switch/1
  Abs/1 -> Relational Operator/2
  Relational Operator/1 -> Switch/2
  Constant/1 -> Switch/3
  Constant2/1 -> Relational Operator/1
  sensor/1 -> Selector/1

== system rlQubeServo/Outer Loop Control/RL_Mode_Select/observation  ==
  sensor : Inport
  Demux : Demux
  Mux : Mux  Inputs=6
  Trigonometric Function : Trigonometry
  Trigonometric Function1 : Trigonometry  Operator=cos
  Trigonometric Function2 : Trigonometry
  Trigonometric Function3 : Trigonometry  Operator=cos
  observation : Outport
  wires:
  Demux/3 -> Mux/5
  Demux/1 -> Trigonometric Function1/1, Trigonometric Function/1
  Trigonometric Function1/1 -> Mux/2
  Trigonometric Function/1 -> Mux/1
  Mux/1 -> observation/1  "observation"
  sensor/1 -> Demux/1
  Trigonometric Function2/1 -> Mux/3
  Trigonometric Function3/1 -> Mux/4
  Demux/2 -> Trigonometric Function3/1, Trigonometric Function2/1
  Demux/4 -> Mux/6

== system rlQubeServo/Outer Loop Control/RL_Mode_Select/reward ==
  sensor : Inport
  action : Inport  Port=2
  isdone_flag : Inport  Port=3
  Add : Sum  Inputs=+++
  Constant : Constant  Value=[0; pi; 0; 0]
  Sum1 : Sum  Inputs=|+-
  change_angle_range : Subsystem
  cost_function : Subsystem
  failure_cost : Subsystem
  success_reward : Subsystem
  reward : Outport
  wires:
  isdone_flag/1 -> failure_cost/1(isdone_flag)
  failure_cost/1(reward) -> Add/3
  success_reward/1(reward) -> Add/1
  cost_function/1(reward) -> Add/2
  action/1 -> cost_function/2(action)
  Add/1 -> reward/1
  Sum1/1 -> change_angle_range/1(In1)
  sensor/1 -> Sum1/2
  Constant/1 -> Sum1/1
  change_angle_range/1(sensor_dif) -> success_reward/1(sensor_dif), cost_function/1(sensor_dif)

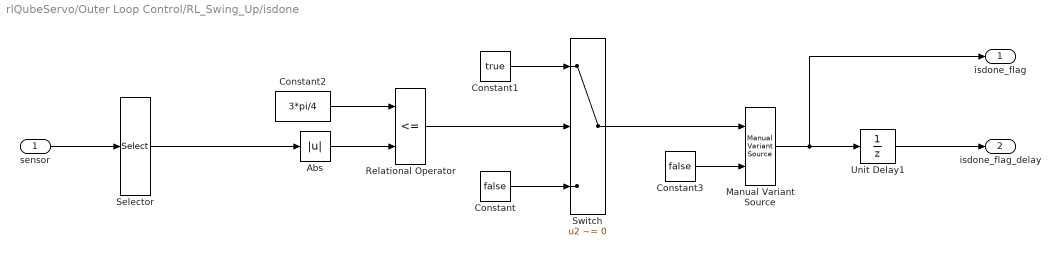
== system rlQubeServo/Outer Loop Control/RL_Swing_Up/isdone ==
  sensor : Inport
  Abs : Abs  SaturateOnIntegerOverflow=off
  Constant : Constant  Value=false
  Constant1 : Constant  Value=true
  Constant2 : Constant  Value=3*pi/4
  Constant3 : Constant  Value=false
  Manual Variant Source : simulink/Signal Routing/Manual Variant Source  NumChoices=2  LabelModeActiveChoice=V_2
  Relational Operator : RelationalOperator  Operator=<=  OutDataTypeStr=boolean  RndMeth=Simplest  InputSameDT=off
  Selector : Selector  InputPortWidth=4  IndexOptions=Index vector (dialog)  Indices=[1]  OutputSizes=1
  Switch : Switch  Criteria=u2 ~= 0  SaturateOnIntegerOverflow=off  InputSameDT=off
  Unit Delay1 : UnitDelay  SampleTime=-1  HasFrameUpgradeWarning=on
  isdone_flag : Outport
  isdone_flag_delay : Outport  Port=2
  wires:
  sensor/1 -> Selector/1
  Constant2/1 -> Relational Operator/1
  Constant/1 -> Switch/3
  Relational Operator/1 -> Switch/2
  Abs/1 -> Relational Operator/2
  Constant1/1 -> Switch/1
  Selector/1 -> Abs/1
  Switch/1 -> Manual Variant Source/1
  Manual Variant Source/1 -> isdone_flag/1, Unit Delay1/1
  Constant3/1 -> Manual Variant Source/2
  Unit Delay1/1 -> isdone_flag_delay/1

== system rlQubeServo/Outer Loop Control/RL_Swing_Up/observation  ==
  sensor : Inport
  Demux : Demux
  Mux : Mux  Inputs=6
  Trigonometric Function : Trigonometry
  Trigonometric Function1 : Trigonometry  Operator=cos
  Trigonometric Function2 : Trigonometry
  Trigonometric Function3 : Trigonometry  Operator=cos
  observation : Outport
  wires:
  Demux/4 -> Mux/6
  Demux/2 -> Trigonometric Function2/1, Trigonometric Function3/1
  Trigonometric Function3/1 -> Mux/4
  Trigonometric Function2/1 -> Mux/3
  sensor/1 -> Demux/1
  Mux/1 -> observation/1  "observation"
  Trigonometric Function/1 -> Mux/1
  Trigonometric Function1/1 -> Mux/2
  Demux/1 -> Trigonometric Function/1, Trigonometric Function1/1
  Demux/3 -> Mux/5

== system rlQubeServo/Outer Loop Control/RL_Swing_Up/reward ==
  sensor : Inport
  action : Inport  Port=2
  isdone_flag : Inport  Port=3
  Add : Sum  Inputs=+++
  Constant : Constant  Value=[0; pi; 0; 0]
  Sum1 : Sum  Inputs=|+-
  change_angle_range : Subsystem
  cost_function : Subsystem
  failure_cost : Subsystem
  success_reward : Subsystem
  reward : Outport
  wires:
  isdone_flag/1 -> failure_cost/1(isdone_flag)
  failure_cost/1(reward) -> Add/3
  success_reward/1(reward) -> Add/1
  cost_function/1(reward) -> Add/2
  action/1 -> cost_function/2(action)
  Add/1 -> reward/1
  Sum1/1 -> change_angle_range/1(In1)
  sensor/1 -> Sum1/2
  Constant/1 -> Sum1/1
  change_angle_range/1(sensor_dif) -> success_reward/1(sensor_dif), cost_function/1(sensor_dif)

== system rlQubeServo/Qube servo/DC Motor model/Sensing ==
  Ideal Rotational Motion Sensor : fl_lib/Mechanical/Mechanical Sensors/Ideal Rotational Motion Sensor  reference=foundation.enum.MeasurementReference.difference  acceleration_port=false  velocity_port=true  position_port=true  wrap_angle=simscape.enum.onoff.off  offset=0 rad
  Mechanical Rotational Reference2 : fl_lib/Mechanical/Rotational Elements/Mechanical Rotational Reference
  PS-Simulink Converter 1 : nesl_utility/PS-Simulink Converter  PhysicalDomain=network_engine_domain  SubClassName=ps_output  LeftPortType=input  RightPortType=output  PseudoPeriodic=off  Frequencies=[]  VectorFormat=1-D array  Unit=inherit  AffineConversion=off
  PS-Simulink Converter 2 : nesl_utility/PS-Simulink Converter  PhysicalDomain=network_engine_domain  SubClassName=ps_output  LeftPortType=input  RightPortType=output  PseudoPeriodic=off  Frequencies=[]  VectorFormat=1-D array  Unit=inherit  AffineConversion=off
  R : PMIOPort  Side=Left
  theta_m : Outport  VectorParamsAs1DForOutWhenUnconnected=off
  omega_m : Outport  Port=2  VectorParamsAs1DForOutWhenUnconnected=off
  wires:
  PS-Simulink Converter 1/1 -> omega_m/1
  PS-Simulink Converter 2/1 -> theta_m/1
  connections:
  PS-Simulink Converter 1/LConn1 -- Ideal Rotational Motion Sensor/RConn2
  Mechanical Rotational Reference2/LConn1 -- Ideal Rotational Motion Sensor/RConn1
  R/RConn1 -- Ideal Rotational Motion Sensor/LConn1
  PS-Simulink Converter 2/LConn1 -- Ideal Rotational Motion Sensor/RConn3

== system rlQubeServo/Qube servo/Pendulum Physical Model/Base ==
  Base : sm_lib/Body Elements/Brick Solid  BrickDimensions=[1 1 1]*10  BrickDimensionsUnits=cm  ExportEntireGeometry=off  InertiaType=CalculateFromGeometry  BasedOnType=Density  Density=1000  DensityUnits=kg/m^3  Mass=1  MassUnits=kg  CenterOfMass=[0 0 0]  CenterOfMassUnits=m  MomentsOfInertia=[1 1 1]  MomentsOfInertiaUnits=kg*m^2  ProductsOfInertia=[0 0 0]  ProductsOfInertiaUnits=kg*m^2  GraphicType=FromGeometry  MarkerShape=Sphere  MarkerSize=10  GraphicVisPropType=SimpleVisualProperties  GraphicDiffuseColor=[0.4 0.4 0.4]  GraphicOpacity=1.0  GraphicSpecularColor=[0.5 0.5 0.5 1.0]  GraphicAmbientColor=[0.15 0.15 0.15 1.0]  GraphicEmissiveColor=[0.0 0.0 0.0 1.0]  GraphicShininess=75  DoExposeReferenceFrame=on  SerializedFrames=<Frames/>
  Rigid Transform : sm_lib/Frames and Transforms/Rigid Transform  RotationMethod=None  FollAlignAxisA=+X  BaseAlignAxisA=+Y  FollAlignAxisB=+Y  BaseAlignAxisB=+Z  RotationStandardAxis=+Z  RotationAngle=0.0  RotationAngleUnits=deg  RotationArbitraryAxis=[0 0 1]  RotationSequenceAxes=FollowerAxes  RotationSequence=XYX  RotationSequenceAngles=[0 0 0]  RotationSequenceAnglesUnits=deg  RotationMatrix=[1 0 0; 0 1 0; 0 0 1]  Quaternion=[1 0 0 0]  TranslationMethod=Cartesian  TranslationCartesianOffset=[-0.016 0 0.051]  TranslationCartesianOffsetUnits=m  TranslationStandardAxis=+Z  TranslationStandardOffset=0  TranslationStandardOffsetUnits=m  TranslationROffset=0  TranslationROffsetUnits=m  TranslationThetaOffset=0  TranslationThetaOffsetUnits=deg  TranslationZOffset=0  TranslationZOffsetUnits=m
  Stopper : sm_lib/Body Elements/Brick Solid  BrickDimensions=[0.01, 0.02, 0.01]  BrickDimensionsUnits=m  ExportEntireGeometry=on  InertiaType=CalculateFromGeometry  BasedOnType=Density  Density=1000  DensityUnits=kg/m^3  Mass=1  MassUnits=kg  CenterOfMass=[0 0 0]  CenterOfMassUnits=m  MomentsOfInertia=[1 1 1]  MomentsOfInertiaUnits=kg*m^2  ProductsOfInertia=[0 0 0]  ProductsOfInertiaUnits=kg*m^2  GraphicType=FromGeometry  MarkerShape=Sphere  MarkerSize=10  GraphicVisPropType=SimpleVisualProperties  GraphicDiffuseColor=[0.5 0.5 0.5]  GraphicOpacity=1.0  GraphicSpecularColor=[0.5 0.5 0.5 1.0]  GraphicAmbientColor=[0.15 0.15 0.15 1.0]  GraphicEmissiveColor=[0.0 0.0 0.0 1.0]  GraphicShininess=75  DoExposeReferenceFrame=on  SerializedFrames=<Frames/>
  Conn1 : PMIOPort  Side=Right
  SCF : PMIOPort  Port=2  Side=Left
  connections:
  Base/RConn1 -- Conn1/RConn1 -- Rigid Transform/LConn1
  Stopper/RConn1 -- Rigid Transform/RConn1
  Stopper/LConn1 -- SCF/RConn1

== system rlQubeServo/Qube servo/Pendulum Physical Model/Encoder ==
  Cylindrical Solid : sm_lib/Body Elements/Cylindrical Solid  CylinderRadius=1.35  CylinderRadiusUnits=cm  CylinderLength=5  CylinderLengthUnits=cm  ExportEntireGeometry=off  InertiaType=CalculateFromGeometry  BasedOnType=Density  Density=3.32e+03  DensityUnits=kg/m^3  Mass=0  MassUnits=kg  CenterOfMass=[0 0 0]  CenterOfMassUnits=m  MomentsOfInertia=[1 1 1]  MomentsOfInertiaUnits=kg*m^2  ProductsOfInertia=[0 0 0]  ProductsOfInertiaUnits=kg*m^2  GraphicType=FromGeometry  MarkerShape=Sphere  MarkerSize=10  GraphicVisPropType=SimpleVisualProperties  GraphicDiffuseColor=[1.0 0.2 0.2]  GraphicOpacity=1.0  GraphicSpecularColor=[0.5 0.5 0.5 1.0]  GraphicAmbientColor=[0.15 0.15 0.15 1.0]  GraphicEmissiveColor=[0.0 0.0 0.0 1.0]  GraphicShininess=75  DoExposeReferenceFrame=on  SerializedFrames=<Frames/>
  Rigid Transform : sm_lib/Frames and Transforms/Rigid Transform  RotationMethod=None  FollAlignAxisA=+X  BaseAlignAxisA=+Y  FollAlignAxisB=+Y  BaseAlignAxisB=+Z  RotationStandardAxis=+Z  RotationAngle=0.0  RotationAngleUnits=deg  RotationArbitraryAxis=[0 0 1]  RotationSequenceAxes=FollowerAxes  RotationSequence=XYX  RotationSequenceAngles=[0 0 0]  RotationSequenceAnglesUnits=deg  RotationMatrix=[1 0 0; 0 1 0; 0 0 1]  Quaternion=[1 0 0 0]  TranslationMethod=Cartesian  TranslationCartesianOffset=[0.015 0 0.02]  TranslationCartesianOffsetUnits=m  TranslationStandardAxis=+Z  TranslationStandardOffset=0  TranslationStandardOffsetUnits=m  TranslationROffset=0  TranslationROffsetUnits=m  TranslationThetaOffset=0  TranslationThetaOffsetUnits=deg  TranslationZOffset=0  TranslationZOffsetUnits=m
  Rigid Transform4 : sm_lib/Frames and Transforms/Rigid Transform  RotationMethod=StandardAxis  FollAlignAxisA=+X  BaseAlignAxisA=+Y  FollAlignAxisB=+Y  BaseAlignAxisB=+Z  RotationStandardAxis=+Y  RotationAngle=90  RotationAngleUnits=deg  RotationArbitraryAxis=[0 0 1]  RotationSequenceAxes=FollowerAxes  RotationSequence=XYX  RotationSequenceAngles=[0 0 0]  RotationSequenceAnglesUnits=deg  RotationMatrix=[1 0 0; 0 1 0; 0 0 1]  Quaternion=[1 0 0 0]  TranslationMethod=None  TranslationCartesianOffset=[0 0 0]  TranslationCartesianOffsetUnits=cm  TranslationStandardAxis=+Z  TranslationStandardOffset=0  TranslationStandardOffsetUnits=cm  TranslationROffset=0  TranslationROffsetUnits=m  TranslationThetaOffset=0  TranslationThetaOffsetUnits=deg  TranslationZOffset=0  TranslationZOffsetUnits=m
  bumper : sm_lib/Curves and Surfaces/Point Cloud  CoordinatesMatrix=[0 0 0]  CoordinatesMatrixUnits=m  GraphicType=MarkerCloud  GraphicSphereRadius=4e-3  GraphicSphereRadiusUnits=m  GraphicVisPropType=SimpleVisualProperties  GraphicDiffuseColor=[0.5 0.5 0.5]  GraphicOpacity=1.0  GraphicSpecularColor=[0.5 0.5 0.5 1.0]  GraphicAmbientColor=[0.15 0.15 0.15 1.0]  GraphicEmissiveColor=[0.0 0.0 0.0 1.0]  GraphicShininess=75
  Conn1 : PMIOPort  Side=Left
  SCF : PMIOPort  Port=2  Side=Right
  connections:
  Rigid Transform4/LConn1 -- Conn1/RConn1
  Rigid Transform/RConn1 -- bumper/LConn1
  Rigid Transform/LConn1 -- Cylindrical Solid/RConn1 -- Rigid Transform4/RConn1
  SCF/RConn1 -- bumper/RConn1

== system rlQubeServo/Qube servo/Pendulum Physical Model/Pendulum ==
  Cylindrical Solid : sm_lib/Body Elements/Cylindrical Solid  CylinderRadius=p_rad  CylinderRadiusUnits=m  CylinderLength=p_length  CylinderLengthUnits=m  ExportEntireGeometry=off  InertiaType=CalculateFromGeometry  BasedOnType=Density  Density=rho_p  DensityUnits=kg/m^3  Mass=1  MassUnits=kg  CenterOfMass=[0 0 0]  CenterOfMassUnits=m  MomentsOfInertia=[1 1 1]  MomentsOfInertiaUnits=kg*m^2  ProductsOfInertia=[0 0 0]  ProductsOfInertiaUnits=kg*m^2  GraphicType=FromGeometry  MarkerShape=Sphere  MarkerSize=10  GraphicVisPropType=SimpleVisualProperties  GraphicDiffuseColor=[1.0 0.0 0.0]  GraphicOpacity=1.0  GraphicSpecularColor=[0.5 0.5 0.5 1.0]  GraphicAmbientColor=[0.15 0.15 0.15 1.0]  GraphicEmissiveColor=[0.0 0.0 0.0 1.0]  GraphicShininess=75  DoExposeReferenceFrame=on  SerializedFrames=<Frames/>
  Rigid Transform : sm_lib/Frames and Transforms/Rigid Transform  RotationMethod=None  FollAlignAxisA=+X  BaseAlignAxisA=+Y  FollAlignAxisB=+Y  BaseAlignAxisB=+Z  RotationStandardAxis=+Z  RotationAngle=0.0  RotationAngleUnits=deg  RotationArbitraryAxis=[0 0 1]  RotationSequenceAxes=FollowerAxes  RotationSequence=XYX  RotationSequenceAngles=[0 0 0]  RotationSequenceAnglesUnits=deg  RotationMatrix=[1 0 0; 0 1 0; 0 0 1]  Quaternion=[1 0 0 0]  TranslationMethod=StandardAxis  TranslationCartesianOffset=[0 0 0]  TranslationCartesianOffsetUnits=m  TranslationStandardAxis=+Z  TranslationStandardOffset=p_length/2 - 0.007  TranslationStandardOffsetUnits=m  TranslationROffset=0  TranslationROffsetUnits=m  TranslationThetaOffset=0  TranslationThetaOffsetUnits=deg  TranslationZOffset=0  TranslationZOffsetUnits=m
  Conn1 : PMIOPort  Side=Left
  connections:
  Conn1/RConn1 -- Rigid Transform/LConn1
  Rigid Transform/RConn1 -- Cylindrical Solid/RConn1

== system rlQubeServo/Qube servo/Pendulum Physical Model/Rod ==
  Cylindrical Solid : sm_lib/Body Elements/Cylindrical Solid  CylinderRadius=rod_rad  CylinderRadiusUnits=m  CylinderLength=rod_length  CylinderLengthUnits=m  ExportEntireGeometry=off  InertiaType=CalculateFromGeometry  BasedOnType=Density  Density=rho_rod  DensityUnits=kg/m^3  Mass=1  MassUnits=kg  CenterOfMass=[0 0 0]  CenterOfMassUnits=m  MomentsOfInertia=[1 1 1]  MomentsOfInertiaUnits=kg*m^2  ProductsOfInertia=[0 0 0]  ProductsOfInertiaUnits=kg*m^2  GraphicType=FromGeometry  MarkerShape=Sphere  MarkerSize=10  GraphicVisPropType=SimpleVisualProperties  GraphicDiffuseColor=[0.8 0.8 0.8]  GraphicOpacity=1.0  GraphicSpecularColor=[0.5 0.5 0.5 1.0]  GraphicAmbientColor=[0.15 0.15 0.15 1.0]  GraphicEmissiveColor=[0.0 0.0 0.0 1.0]  GraphicShininess=75  DoExposeReferenceFrame=on  SerializedFrames=<Frames/>
  Conn1 : PMIOPort  Side=Left
  connections:
  Conn1/RConn1 -- Cylindrical Solid/RConn1

== system rlQubeServo/Qube servo/Pendulum Physical Model/stopper ==
  stopper_off : Subsystem  VariantControl=Choice_Qube_Stopper_Off
  stopper_on : Subsystem  VariantControl=Choice_Qube_Stopper_On
  Conn1 : PMIOPort  Side=Left
  Conn2 : PMIOPort  Port=2  Side=Right

== system rlQubeServo/Outer Loop Control/RL_Mode_Select/reward/change_angle_range ==
  In1 : Inport
  Demux : Demux
  Mux : Mux
  change_angle_range : Subsystem
  change_angle_range1 : Subsystem
  mod_2pi : Subsystem
  mod_2pi1 : Subsystem
  sensor_dif : Outport
  wires:
  mod_2pi1/1(Out_angle) -> change_angle_range1/1(In_angle)
  mod_2pi/1(Out_angle) -> change_angle_range/1(In_angle)
  Mux/1 -> sensor_dif/1
  Demux/4 -> Mux/4
  Demux/3 -> Mux/3
  change_angle_range1/1(Out_angle) -> Mux/2
  change_angle_range/1(Out_angle) -> Mux/1
  In1/1 -> Demux/1
  Demux/1 -> mod_2pi/1(In_angle)
  Demux/2 -> mod_2pi1/1(In_angle)

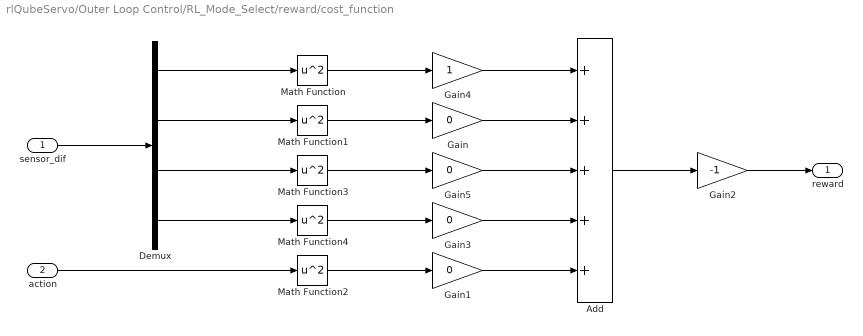
== system rlQubeServo/Outer Loop Control/RL_Mode_Select/reward/cost_function ==
  sensor_dif : Inport
  action : Inport  Port=2
  Add : Sum  Inputs=+++++
  Demux : Demux
  Gain{,1,3,5} (4 alike) : Gain  Gain=0
  Gain2 : Gain  Gain=-1
  Gain4 : Gain
  Math Function{,1..4} (5 alike) : Math  Operator=square
  reward : Outport
  wires:
  Math Function4/1 -> Gain3/1
  Gain4/1 -> Add/1
  Gain/1 -> Add/2
  Gain5/1 -> Add/3
  Gain3/1 -> Add/4
  Gain1/1 -> Add/5
  Gain2/1 -> reward/1
  Add/1 -> Gain2/1
  sensor_dif/1 -> Demux/1
  Demux/4 -> Math Function4/1
  Demux/3 -> Math Function3/1
  Demux/2 -> Math Function1/1
  Math Function1/1 -> Gain/1
  Math Function3/1 -> Gain5/1
  action/1 -> Math Function2/1
  Demux/1 -> Math Function/1
  Math Function/1 -> Gain4/1
  Math Function2/1 -> Gain1/1
